simulink model "TTQC_ProcessTransTrqReq_Error"  (Simulink 7.8)
settings: Solver=FixedStepDiscrete  StartTime=0.0  StopTime=50.0  FixedStep=0.0001  RelTol=1e-3
libraries: ChryslerLib x3
settings Model: Creator=chrysler2  LastModifiedBy=monika
settings DebuggingCC: CheckSSInitialOutputMsg=off  MergeDetectMultiDrivingBlocksExec=error

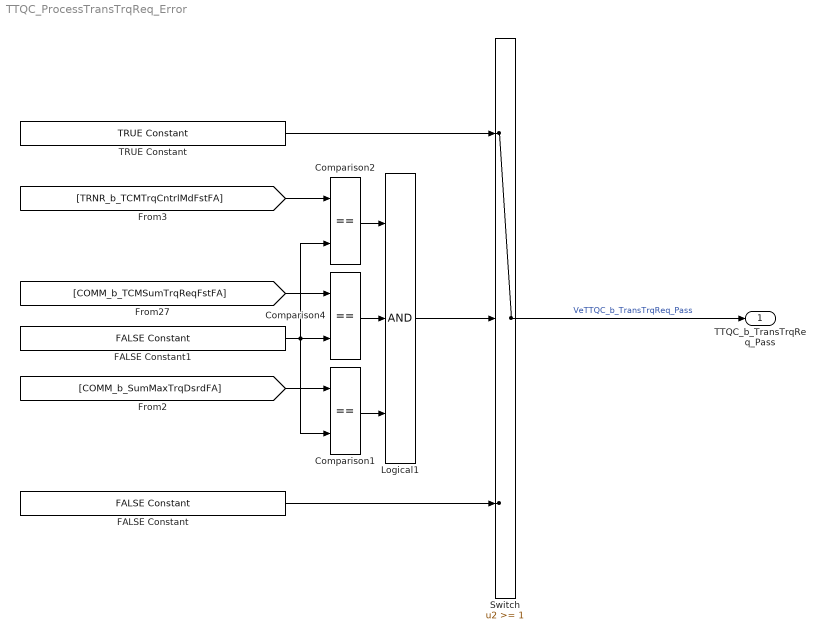
== system TTQC_ProcessTransTrqReq_Error ==
  Comparison1 : RelationalOperator  Operator===  OutDataTypeStr=boolean
  Comparison2 : RelationalOperator  Operator===  OutDataTypeStr=boolean
  Comparison4 : RelationalOperator  Operator===  OutDataTypeStr=boolean
  FALSE Constant : ChryslerLib/Parameters & Constants/FALSE Constant
  FALSE Constant1 : ChryslerLib/Parameters & Constants/FALSE Constant
  Logical1 : Logic  Inputs=3  OutDataTypeStr=boolean
  Switch : Switch  Threshold=1  RndMeth=Zero  InputSameDT=on
      settings: AttributesFormatString=Threshold=%<Threshold>
  TRUE Constant : ChryslerLib/Parameters & Constants/TRUE Constant
  TTQC_b_TransTrqReq_Pass : Outport
  wires:
  Comparison1/1 -> Logical1/3
  Logical1/1 -> Switch/2
  [COMM_b_SumMaxTrqDsrdFA] -> Comparison1/1
  [COMM_b_TCMSumTrqReqFstFA] -> Comparison4/1
  Switch/1 -> TTQC_b_TransTrqReq_Pass/1  "VeTTQC_b_TransTrqReq_Pass"
  TRUE Constant/1 -> Switch/1
  FALSE Constant1/1 -> Comparison1/2, Comparison4/2, Comparison2/2
  Comparison4/1 -> Logical1/2
  FALSE Constant/1 -> Switch/3
  Comparison2/1 -> Logical1/1
  [TRNR_b_TCMTrqCntrlMdFstFA] -> Comparison2/1
